simulink model "control_vectorial_dc"  (R2024b)
settings: Solver=ode14x  StartTime=0.0  StopTime=1  FixedStep=1e-6  MaxStep=1e-5  MinStep=1e-7  RelTol=1e-4  EnableMultiTasking=on
model workspace (MAT data in the model file):
  I_speed = 0.006
  P_flux = 0.72
  P_speed = 1.04
  P_torque = 0.72
  w = 2000
libraries: ee_lib x10, nesl_utility x7, fl_lib x5, eePwmGenerator x1, eeDcCurrentController x1, slpidlib x1
Description:
  | Field-Oriented Control al unui motor de tip Brushless DC, implementat cu uController, generator de PWM si driver.
settings Model: SimulationMode=accelerator  Creator=radu  LastModifiedBy=radu
settings SolverCC: PositivePriorityOrder=on  AutoInsertRateTranBlk=on
settings OptimizationCC: DefaultParameterBehavior=Inlined  EnhancedBackFolding=on  PassReuseOutputArgsThreshold=0  MaxStackSize=64  OptimizeBlockOrder=speed  DifferentSizesBufferReuse=on  OptimizationCustomize=off
settings DebuggingCC: ParameterTunabilityLossMsg=error
settings HardwareCC: HardwareBoardFeatureSet=SoCBlockset
settings ModelReferenceCC: ModelReferenceNumInstancesAllowed=Single
settings SFSimCC: MATLABDynamicMemAlloc=off
settings CodeAppCC: ForceParamTrailComments=on  OperatorAnnotations=on
settings GRTTargetCC: TargetLangStandard=C89/C90 (ANSI)

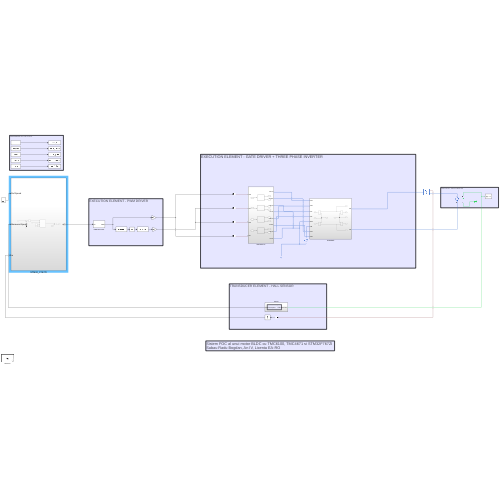
[thumbnail: Simulink's stored preview of the top-level diagram]
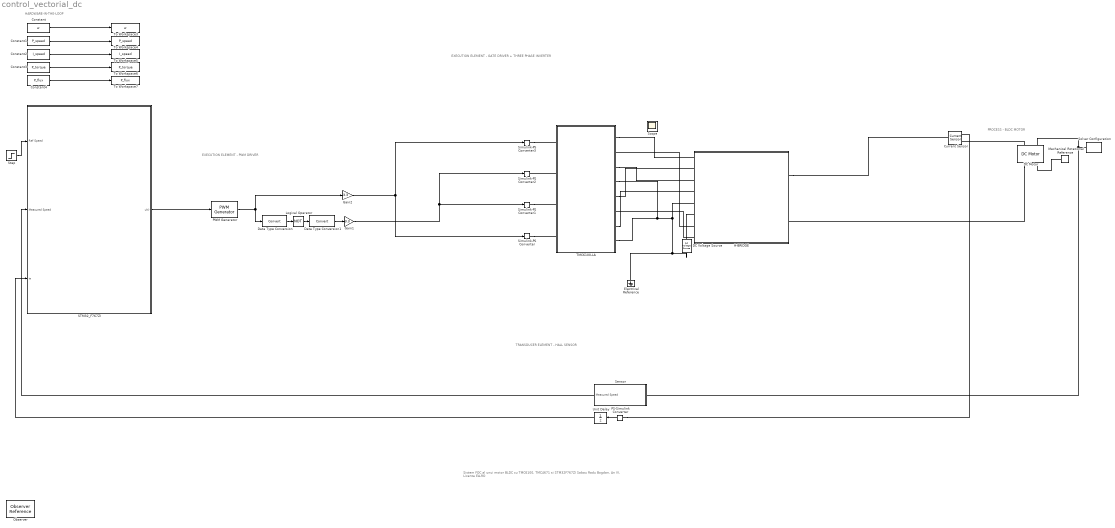
== system control_vectorial_dc ==
  note: HARDWARE-IN-THE-LOOP
  note: EXECUTION ELEMENT - PWM DRIVER
  note: PROCESS - BLDC MOTOR
  note: Sistem FOC al unui motor BLDC cu TMC6100, TMC4671 si STM32F767ZI
      | Sabau Radu Bogdan, An IV, Licenta EA-RO
  note: TRANSDUCER ELEMENT - HALL SENSOR
  note: EXECUTION ELEMENT - GATE DRIVER + THREE PHASE INVERTER
  Constant : Constant  Value=w
  Constant1 : Constant  Value=P_speed
  Constant2 : Constant  Value=I_speed
  Constant3 : Constant  Value=P_torque
  Constant4 : Constant  Value=P_flux
  Current Sensor : fl_lib/Electrical/Electrical Sensors/Current Sensor
  DC Motor : ee_lib/Electromechanical/Brushed Motors/DC Motor  field_option=ee.enum.field_option.pm  Rf=100 Ohm  Lf=1 H  Laf=0.15 H  If0=0 A  parameterization=ee.enum.dcparam_option.load_speed  Ra=3.9 Ohm  La=565e-6 H  emf_or_torque=ee.enum.emf_or_torque.kv  Kv=0.072e-3 V/rpm  Ki=6.876e-4 N*m/A  T_stall=0.24e-3 N*m  w_max=14974 rpm  w_rated=12850 rpm  P_rated=9.504 W  V_rated=12 V  lam_param=ee.enum.lam_param.damping  i_noload=0 A  V_i_noload=1.5 V  J=1e-6 kg*m^2  lam=5e-6 N*m*s/rad  speed0=0 rpm  t_fault_armature=1 s  t_fault_field=1 s  fault_action=simscape.enum.assert.action.none  alpha=3.93e-3 1/K  Tmeas=25 degC  thermal_mass=100 J/K  initial_temperature=25 degC
  DC Voltage Source : ee_lib/Additional Components/SPICE Sources/DC Voltage Source  DC=12 V
  Data Type Conversion : DataTypeConversion  SaturateOnIntegerOverflow=off  RndMeth=Floor
  Data Type Conversion1 : DataTypeConversion  SaturateOnIntegerOverflow=off  RndMeth=Floor
  Electrical Reference : fl_lib/Electrical/Electrical Elements/Electrical Reference
  Gain1 : Gain  Gain=3.3  OutDataTypeStr=double
  Gain2 : Gain  Gain=3.3  OutDataTypeStr=double
  H-BRIDGE : Subsystem
  Logical Operator : Logic  Operator=NOT  AllPortsSameDT=off  OutDataTypeStr=boolean
  Mechanical Rotational Reference : fl_lib/Mechanical/Rotational Elements/Mechanical Rotational Reference
  Observer : ObserverReference  ObserverModelName=control_vectorial_dc_v2_Observer1
  PS-Simulink Converter : nesl_utility/PS-Simulink Converter  PhysicalDomain=network_engine_domain  SubClassName=ps_output  LeftPortType=input  RightPortType=output  PseudoPeriodic=off  Frequencies=[]  VectorFormat=inherit  Unit=inherit  AffineConversion=off
  PWM Generator : eePwmGenerator/PWM Generator  CarrCount=Up  Tper=0.00002  Tdelay=0  Ts=1e-6
  STM32_F767ZI : Subsystem
  Sensor : Subsystem
  Simulink-PS Converter{,1..3} (4 alike) : nesl_utility/Simulink-PS Converter  PhysicalDomain=network_engine_domain  SubClassName=ps_input  LeftPortType=input  RightPortType=output  PseudoPeriodic=off  Frequencies=[]  NoiseDistribution=none  NoiseParameters=[]  Unit=1  AffineConversion=off  FilteringAndDerivatives=provide  SimscapeFilterOrder=1  InputFilterTimeConstant=0.001  UdotUserProvided=0
  Solver Configuration : nesl_utility/Solver Configuration  PhysicalDomain=network_engine_domain  SubClassName=solver  LeftPortType=input  RightPortType=generic  Tones=[]  Harmonics=[]  SimulateNoise=off  Profile=off  UseLocalSampling=off  EnableSwitchedLinearOptims=on  FrequencyDomain=off  UseCCode=off  RelTol=0.001  AbsTol=0.001  MinStep=1e-09  ToWorkspace=off  RevertToSquareIcSolve=off  NumHomotopyIterations=100  PhasorMode=off  PhasorModeNumHarmonics=1  ConsistencySolver=NEWTON_XTOL_AFTER_FTOL  IndexReductionMethod=DerivativeReplacement  DoDC=off  ResidualTolerance=1e-09  ConsistencyTolSource=GLOBAL  ConsistencyAbsTol=0.001  ConsistencyRelTol=0.001  ConsistencyTolFactor=1e-4  UseLocalSolver=on  LocalSolverChoice=NE_TRAPEZOIDAL_ADVANCER  ResolveIndetEquations=on  FunctionEvalNumThread=1  LocalSolverSampleTime=1e-6  DoFixedCost=on  MaxNonlinIter=3  MaxModeIter=2  ComputeImpulses=off  ImpulseIterations=2  LinearAlgebra=auto  LinearAlgebraNumThread=0  EquationFormulation=NE_TIME_EF  DelaysMemoryBudget=1024  AutomaticFiltering=on  FilteringTimeConstant=0.001  PartitionStorageMethod=AS_NEEDED  PartitionMemoryBudget=1024  PartitionMethod=ROBUST  MultibodyUseLocalSolver=off  MultibodyLocalSolverChoice=ODE1  MultibodyLocalSolverSampleTime=0.001
  Step : Step  Time=0  After=2500  SampleTime=1e-6
  TMC6100-LA : Subsystem
  To Workspace3 : ToWorkspace  VariableName=w  SaveFormat=Timeseries  SampleTime=-1
  To Workspace4 : ToWorkspace  VariableName=P_speed  SaveFormat=Timeseries  SampleTime=-1
  To Workspace5 : ToWorkspace  VariableName=I_speed  SaveFormat=Timeseries  SampleTime=-1
  To Workspace6 : ToWorkspace  VariableName=P_torque  SaveFormat=Timeseries  SampleTime=-1
  To Workspace7 : ToWorkspace  VariableName=P_flux  SaveFormat=Timeseries  SampleTime=-1
  Unit Delay : UnitDelay  SampleTime=-1  HasFrameUpgradeWarning=on
  Scope : Scope
  wires:
  Sensor/1(Measured Speed) -> STM32_F767ZI/2(Measured Speed)
  Step/1 -> STM32_F767ZI/1(Ref Speed)
  Constant/1 -> To Workspace3/1
  Constant4/1 -> To Workspace7/1
  Constant2/1 -> To Workspace5/1
  Constant3/1 -> To Workspace6/1
  Constant1/1 -> To Workspace4/1
  PWM Generator/1 -> Gain2/1, Data Type Conversion/1
  STM32_F767ZI/1(u(t)) -> PWM Generator/1
  Data Type Conversion/1 -> Logical Operator/1
  Data Type Conversion1/1 -> Gain1/1
  Logical Operator/1 -> Data Type Conversion1/1
  PS-Simulink Converter/1 -> Unit Delay/1
  Unit Delay/1 -> STM32_F767ZI/3(ia)
  Gain1/1 -> Simulink-PS Converter1/1, Simulink-PS Converter2/1
  Gain2/1 -> Simulink-PS Converter/1, Simulink-PS Converter3/1
  connections:
  Sensor/LConn1 -- Solver Configuration/RConn1 -- DC Motor/LConn2
  Mechanical Rotational Reference/LConn1 -- DC Motor/RConn2
  TMC6100-LA/RConn1 -- H-BRIDGE/LConn1
  TMC6100-LA/RConn3 -- H-BRIDGE/LConn3
  TMC6100-LA/RConn5 -- H-BRIDGE/LConn2
  TMC6100-LA/RConn7 -- H-BRIDGE/LConn4
  TMC6100-LA/RConn8 -- TMC6100-LA/RConn4 -- DC Voltage Source/RConn1 -- Electrical Reference/LConn1 -- H-BRIDGE/LConn5
  H-BRIDGE/LConn6 -- DC Voltage Source/LConn1
  Simulink-PS Converter3/RConn1 -- TMC6100-LA/LConn1
  TMC6100-LA/LConn2 -- Simulink-PS Converter2/RConn1
  Simulink-PS Converter1/RConn1 -- TMC6100-LA/LConn3
  Simulink-PS Converter/RConn1 -- TMC6100-LA/LConn4
  H-BRIDGE/LConn7 -- TMC6100-LA/RConn2
  H-BRIDGE/LConn8 -- TMC6100-LA/RConn6
  DC Motor/RConn1 -- H-BRIDGE/RConn2
  DC Motor/LConn1 -- Current Sensor/RConn2
  H-BRIDGE/RConn1 -- Current Sensor/LConn1
  PS-Simulink Converter/LConn1 -- Current Sensor/RConn1

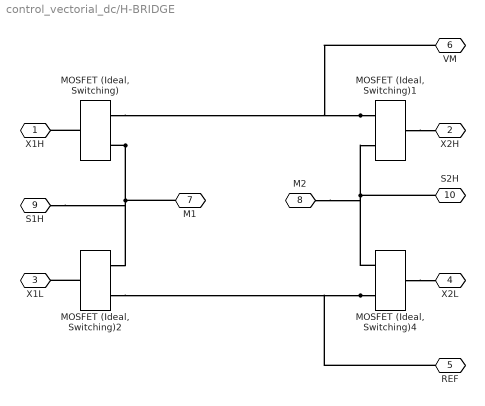
== system control_vectorial_dc/H-BRIDGE ==
  MOSFET (Ideal, Switching){,1..2,4} (4 alike) : ee_lib/Semiconductors & Converters/MOSFET (Ideal, Switching)  port_option=ee.enum.controlport.elec  Rds=0.0021 Ohm  Goff=140 1/Ohm  Vth=3 V  diode_param=ee.enum.semiconductors.protectionDiode.nodynamics  diode_Vf=0.1 V  diode_Ron=0.001 Ohm  diode_Goff=1e-5 1/Ohm  diode_C=50e-9 F  diode_iRM=-235 A  diode_iF=300 A  diode_idot=-50 A/us  diode_trr_param=ee.enum.converters.diodeReverseParam.trr_factor  diode_trr_factor=3  diode_trr=15 us  diode_Qrr=1500 s*uA  ids_specify=off  ids_priority=None  ids=0 A  ids_nominal_specify=off  ids_nominal_value=1  ids_nominal_unit=A  vds_specify=off  vds_priority=None  vds=0 V  vds_nominal_specify=off  vds_nominal_value=1  vds_nominal_unit=V  vgs_specify=off  vgs_priority=None  vgs=0 V  vgs_nominal_specify=off  vgs_nominal_value=1  vgs_nominal_unit=V  thermal_loss_option=ee.enum.converters.thermalLossOption.constantvalues  Von_data=[0, 1.8, 3.2, 6, 10, 16; 0, 2, 5.5, 9.5, 15, 25] V  Tj=[298.15, 448.15] K  Iout_data=[0, 20, 40, 60, 80, 100] A  Eon_data=[0, 55.04, 124.57, 235.53, 362.12; 0, 71.25, 161.25, 304.88, 468.75] * 1e-6 J  Eoff_data=[0, 18, 30, 56.1, 76.5; 0, 22.5, 37.5, 70.13, 95.63] * 1e-6 J  Eon_data_3D=[zeros(2, 5, 3)] J  Eoff_data_3D=[zeros(2, 5, 3)] J  Tj_loss=[298.15, 448.15] K  Iout_data_loss=[0, 10, 20, 30, 40] A  tabulateWithVds=false  Vds_loss=[0, 150, 300] V  Eon_scalar=22.86e-3 J  Eoff_scalar=17.14e-3 J  Voff=300 V  Iout_scalar=600 A  useCurrentFromPreviousCycle=false  useVoltageFromPreviousCycle=false  diodeModelType=ee.enum.converters.diodeModelType.pwl  diodeTableType=ee.enum.diode.tableType.IfMat  diode_ReverseIVType=ee.enum.diode.diodeReverseIV.constant  diode_IfMat=[.07, .12, .19, 1.75, 4.24, 7.32, 11.2; .16, .3, .72, 2.14, 4.02, 6.35, 9.12] A  diode_VfMat=[.9, 1.15, 1.25, 1.5, 1.75, 2.17, 2.6, 2.85; .58, .68, .75, 1.1, 1.38, 1.77, 2.27, 2.7] V  diode_TjVec=[25, 125] degC  diode_VfVec=[.5, .7, .9, 1.3, 1.7, 2.1, 2.5] V  diode_IfVec=[.1, .2, .5, 1, 2, 4, 7, 10] A  diode_IrMat=[1e-06, 2e-06, 5e-06, 1e-05, 2.5e-05, 5e-05, .0001; 2e-06, 5e-06, 1e-05, 4e-05, 8e-05, .0002, .0005] A  diode_VrMat=[10, 100, 200, 250, 300, 325, 350; 10, 70, 160, 220, 270, 300, 320] V  diode_VrVec=[10, 20, 40, 50, 70, 80, 100] V  diode_IrVec=[1e-06, 2e-06, 5e-06, 1e-05, 2e-05, 5e-05, .0001] A  diode_Vr=-600 V  diode_Ls=150 nH  diode_Erec=0.03 J  diode_rec_loss_model=ee.enum.diode.reverseRecoveryModel.fixed  diode_ErecVal=0 J  diode_scaleWithIandV=true  diode_ErecMat=zeros(2, 3) J  diode_TjrecVec=[298.15, 398.15] K  diode_IfrecVec=[.1, 1, 10] A  diode_IrecVal=10 A  diode_VrecVal=10 V  diode_tFilter=1 / 1000 / 100 s  separateThermalPortForDiode=false  thermal_network_parameterization=ee.enum.thermalNetworkTopology.external  Rth=[.03, .2] K/W  Rth_Cauer=[.03, .1, .2] K/W  Rth_Foster=[.08, .14, .22, .16] K/W  thermal_mass_parameterization=ee.enum.thermalNetwork.timeconstant  thermal_mass=[3, 25] J/K  thermal_mass_Cauer=[3, 10, 25] J/K  thermal_mass_Foster=[.001, .005, .05, .5] J/K  thermal_time_constant=[.1, 5] s  thermal_time_constant_Cauer=[.1, 1, 5] s  thermal_time_constant_Foster=[7e-05, .0007, .01, .08] s  thermal_mass_initial_temperatures=[25, 25] degC  thermal_mass_initial_temperatures_Cauer=[25, 25, 25] degC  junction_thermal_mass=0.1 J/K  Tvec_initial_Foster=[25, 25, 25, 25] degC  RthDiode=[.03, .2] K/W  RthCauerDiode=[.03, .1, .2] K/W  RthFosterDiode=[.03, .2] K/W  thermalMassDiode=[3, 25] J/K  thermalMassCauerDiode=[3, 10, 25] J/K  thermalMassFosterDiode=[33, 50] J/K  thermalTauDiode=[.1, 5] s  thermalTauCauerDiode=[.1, 1, 5] s  thermalTauFosterDiode=[1, 10] s  thermalMassInitTempDiode=[25, 25] degC  thermalMassInitTempCauerDiode=[25, 25, 25] degC  junctionthermalMassDiode=0.1 J/K  TVecInitialFosterDiode=[25, 25, 25, 25] degC  no_thermal_network=0  mosfet_junction_temperature_specify=off  mosfet_junction_temperature_priority=None  mosfet_junction_temperature=25 degC  mosfet_junction_temperature_nominal_specify=off  mosfet_junction_temperature_nominal_value=1  mosfet_junction_temperature_nominal_unit=degC  diode_junction_temperature_specify=off  diode_junction_temperature_priority=None  diode_junction_temperature=25 degC  diode_junction_temperature_nominal_specify=off  diode_junction_temperature_nominal_value=1  diode_junction_temperature_nominal_unit=degC  Qj_specify=off  Qj_priority=None  Qj=0 W  Qj_nominal_specify=off  Qj_nominal_value=1  Qj_nominal_unit=W  accumulatedSwitchingLosses_specify=off  accumulatedSwitchingLosses_priority=None  accumulatedSwitchingLosses=0 J
      settings: InternalSimscapePortConfiguration="{\"Bottom\":[],\"Left\":[{\"id\":\"G_elec\",\"label\":\"\",\"type\":\"foundation.electrical.electrical\"}],\"Right\":[{\"id\":\"D\",\"label\":\"\",\"type\":\"foundation.electrical.electrical\"},{\"id\":\"S\",\"label\":\"\",\"type\":\"foundation.electrical.electrical\"}],\"Top\":[]}"
  X1H : PMIOPort  Side=Left
  X2H : PMIOPort  Port=2  Side=Left
  X1L : PMIOPort  Port=3  Side=Left
  X2L : PMIOPort  Port=4  Side=Left
  REF : PMIOPort  Port=5  Side=Left
  VM : PMIOPort  Port=6  Side=Left
  M1 : PMIOPort  Port=7  Side=Right
  M2 : PMIOPort  Port=8  Side=Right
  S1H : PMIOPort  Port=9  Side=Left
  S2H : PMIOPort  Port=10  Side=Left
  connections:
  "MOSFET (Ideal, Switching)"/RConn2 -- S1H/RConn1 -- "MOSFET (Ideal, Switching)2"/RConn1 -- M1/RConn1
  "MOSFET (Ideal, Switching)4"/LConn1 -- X2L/RConn1
  "MOSFET (Ideal, Switching)4"/RConn2 -- "MOSFET (Ideal, Switching)2"/RConn2 -- REF/RConn1
  "MOSFET (Ideal, Switching)2"/LConn1 -- X1L/RConn1
  "MOSFET (Ideal, Switching)"/LConn1 -- X1H/RConn1
  "MOSFET (Ideal, Switching)1"/RConn1 -- "MOSFET (Ideal, Switching)"/RConn1 -- VM/RConn1
  "MOSFET (Ideal, Switching)1"/LConn1 -- X2H/RConn1
  "MOSFET (Ideal, Switching)4"/RConn1 -- M2/RConn1 -- S2H/RConn1 -- "MOSFET (Ideal, Switching)1"/RConn2

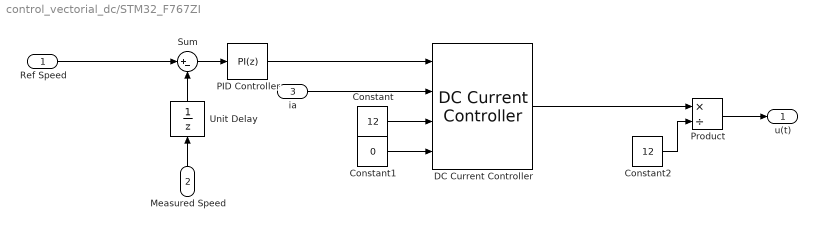
== system control_vectorial_dc/STM32_F767ZI ==
  Ref Speed : Inport
  Measured Speed : Inport  Port=2
  ia : Inport  Port=3
  Constant : Constant  Value=12
  Constant1 : Constant  Value=0
  Constant2 : Constant  Value=12
  DC Current Controller : eeDcCurrentController/DC Current Controller  Kp=1  Ki=1  Kaw=1  VoltLim=Positive and negative voltage  Ts=-1  Tsd=0.001  ActZC=off
      settings: LibrarySourceBlock=|
      | ee_sl_lib/General Machine
      | Control/DC Current Controller
  PID Controller : slpidlib/PID Controller  Controller=PI  Form=Parallel  TimeDomain=Discrete-time  UseExternalTs=off  SampleTime=1e-6  IntegratorMethod=Backward Euler  FilterMethod=Forward Euler  ControllerParametersSource=internal  P=P_speed  I=I_speed  UseKiTs=off  D=1  UseExternalDerivativeSource=off  N=100  UseFilter=on  TunerSelectOption=Transfer Function Based (PID Tuner App)  InitialConditionSource=internal  InitialConditionForIntegrator=0  InitialConditionForFilter=0  DifferentiatorICPrevScaledInput=0  ExternalReset=none  TrackingMode=off  Kt=1  LimitOutput=on  SatLimitsSource=internal  UpperSaturationLimit=15000  LowerSaturationLimit=-15000  LinearizeAsGain=on  AntiWindupMode=none  Kb=1  LimitIntegrator=off  UpperIntegratorSaturationLimit=inf  LowerIntegratorSaturationLimit=-inf  POutMin=[]  POutMax=[]  IOutMin=[]  IOutMax=[]  DOutMin=[]  DOutMax=[]  NOutMin=[]  NOutMax=[]  SumOutMin=[]  SumOutMax=[]  SaturationOutMin=[]  SaturationOutMax=[]  PParamMin=[]  PParamMax=[]  IParamMin=[]  IParamMax=[]  DParamMin=[]  DParamMax=[]  NParamMin=[]  NParamMax=[]  KbParamMin=[]  KbParamMax=[]  KtParamMin=[]  KtParamMax=[]  KbOutMin=[]  KbOutMax=[]  KtOutMin=[]  KtOutMax=[]  IntegratorOutMin=[]  IntegratorOutMax=[]  FilterOutMin=[]  FilterOutMax=[]  SumI1OutMin=[]  SumI1OutMax=[]  SumI2OutMin=[]  SumI2OutMax=[]  SumI3OutMin=[]  SumI3OutMax=[]  SumI4OutMin=[]  SumI4OutMax=[]  SumDOutMin=[]  SumDOutMax=[]  DifferentiatorOutMin=[]  DifferentiatorOutMax=[]  FilterDiffOutCoefMin=[]  FilterDiffOutCoefMax=[]  ReciprocalOutMin=[]  ReciprocalOutMax=[]  SumDenOutMin=[]  SumDenOutMax=[]  SumNumOutMin=[]  SumNumOutMax=[]  DivideOutMin=[]  DivideOutMax=[]  UdiffTsProdOutMin=[]  UdiffTsProdOutMax=[]  NTsProdOutMin=[]  NTsProdOutMax=[]  UintegralTsProdOutMin=[]  UintegralTsProdOutMax=[]  UngainTsProdOutMin=[]  UngainTsProdOutMax=[]  ClampingZeroOutDataTypeStr=Inherit: Inherit via back propagation  ClampingZeroOutMin=[]  ClampingZeroOutMax=[]  FilterDenConstantOutDataTypeStr=Inherit: Inherit via back propagation  FilterDenConstantOutMin=[]  FilterDenConstantOutMax=[]  PCopyOutDataTypeStr=Inherit: Inherit via back propagation  PCopyOutMin=[]  PCopyOutMax=[]  NCopyOutDataTypeStr=Inherit: Inherit via back propagation  NCopyOutMin=[]  NCopyOutMax=[]  IntegratorContinuousStateAttributes=''  IntegratorStateMustResolveToSignalObject=off  IntegratorRTWStateStorageClass=Auto  FilterContinuousStateAttributes=''  FilterStateMustResolveToSignalObject=off  FilterRTWStateStorageClass=Auto  ParallelPVariant=InternalParameters  IdealPVariant=Disabled  IVariant=InternalParameters  DVariant=Disabled  IntegratorVariant=Discrete  SatVariant=Enabled  AWVariant=Passthrough  PCopyVariant=Disabled  TRVariant=Disabled  FdbkBlocksVariant=Forward  IdealPFdbkVariant=Disabled  SatFdbkVariant=Disabled  DerivativeFilterVariant=Disabled  NVariant=Disabled  NCopyVariant=Disabled_SignalSpec  FilterICVariant=Disabled  IntegratorICVariant=InternalICs  ExternalResetVariant=Disabled  TRSumVariant=Passthrough  SumFdbkVariant=Disabled  SumVariant=Sum_PI  TsampFilterVariant=InternalTs  TsampNgainVariant=Passthrough  TsampIntegralVariant=Disabled_SignalSpec  ExternalSaturationOutDataTypeStr=Inherit: Same as second input  DerivativeSourceVariant=Disabled  PreIntVariant=InternalPreInt
  Product : Product  Inputs=*/
  Sum : Sum  Inputs=|+-
  Unit Delay : UnitDelay  SampleTime=1e-5  HasFrameUpgradeWarning=on
  u(t) : Outport
  wires:
  Sum/1 -> PID Controller/1
  Ref Speed/1 -> Sum/1
  Unit Delay/1 -> Sum/2
  Measured Speed/1 -> Unit Delay/1
  Product/1 -> u(t)/1
  Constant2/1 -> Product/2
  Constant1/1 -> DC Current Controller/4
  Constant/1 -> DC Current Controller/3
  DC Current Controller/1 -> Product/1
  ia/1 -> DC Current Controller/2
  PID Controller/1 -> DC Current Controller/1

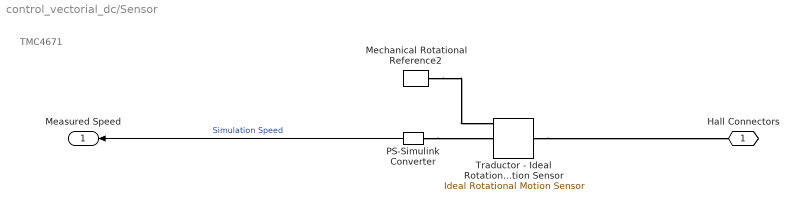
== system control_vectorial_dc/Sensor ==
  note: TMC4671
  Mechanical Rotational Reference2 : fl_lib/Mechanical/Rotational Elements/Mechanical Rotational Reference
  PS-Simulink Converter : nesl_utility/PS-Simulink Converter  PhysicalDomain=network_engine_domain  SubClassName=ps_output  LeftPortType=input  RightPortType=output  PseudoPeriodic=off  Frequencies=[]  VectorFormat=inherit  Unit=rpm  AffineConversion=off
  Traductor - Ideal Rotational Motion Sensor : fl_lib/Mechanical/Mechanical Sensors/Ideal Rotational Motion Sensor  reference=foundation.enum.MeasurementReference.difference  acceleration_port=false  velocity_port=true  position_port=true  wrap_angle=false  offset=0 deg
  Hall Connectors : PMIOPort  Side=Left
  Measured Speed : Outport
  wires:
  PS-Simulink Converter/1 -> Measured Speed/1  "Simulation Speed"
  connections:
  PS-Simulink Converter/LConn1 -- Traductor - Ideal Rotational Motion Sensor/RConn2
  Mechanical Rotational Reference2/LConn1 -- Traductor - Ideal Rotational Motion Sensor/RConn1
  Traductor - Ideal Rotational Motion Sensor/LConn1 -- Hall Connectors/RConn1

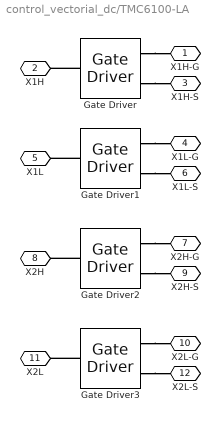
== system control_vectorial_dc/TMC6100-LA ==
  Gate Driver{,1..3} (4 alike) : ee_lib/Semiconductors & Converters/Gate Driver  port_option=ee.enum.controlport.ps  uHigh=2.0 V  uLow=0.8 V  uHighValue=2.31  uLowValue=0.99  vHigh=12 V  vLow=0 V  tHigh=85 ns  tLow=85 ns  parameterization=ee.enum.semiconductors.gateDriverParam.riseAndFallTimes  rHigh=2 Ohm  rLow=2 Ohm  tRise=10 ns  tFall=10 ns  cLoad=10 nF  t_fault=1 s  ZonTime_specify=off  ZonTime_priority=None  ZonTime=0 s  ZoffTime_specify=off  ZoffTime_priority=None  ZoffTime=0 s
      settings: InternalSimscapePortConfiguration="{\"Bottom\":[],\"Left\":[{\"id\":\"u\",\"label\":\"u\",\"type\":\"input\"}],\"Right\":[{\"id\":\"G\",\"label\":\"G\",\"type\":\"foundation.electrical.electrical\"},{\"id\":\"S\",\"label\":\"S\",\"type\":\"foundation.electrical.electrical\"}],\"Top\":[]}"
  X1H-G : PMIOPort  Side=Right
  X1H : PMIOPort  Port=2  Side=Left
  X1H-S : PMIOPort  Port=3  Side=Right
  X1L-G : PMIOPort  Port=4  Side=Right
  X1L : PMIOPort  Port=5  Side=Left
  X1L-S : PMIOPort  Port=6  Side=Right
  X2H-G : PMIOPort  Port=7  Side=Right
  X2H : PMIOPort  Port=8  Side=Left
  X2H-S : PMIOPort  Port=9  Side=Right
  X2L-G : PMIOPort  Port=10  Side=Right
  X2L : PMIOPort  Port=11  Side=Left
  X2L-S : PMIOPort  Port=12  Side=Right
  connections:
  Gate Driver2/LConn1 -- X2H/RConn1
  Gate Driver1/LConn1 -- X1L/RConn1
  Gate Driver1/RConn1 -- X1L-G/RConn1
  Gate Driver1/RConn2 -- X1L-S/RConn1
  Gate Driver2/RConn1 -- X2H-G/RConn1
  Gate Driver/RConn2 -- X1H-S/RConn1
  Gate Driver3/LConn1 -- X2L/RConn1
  Gate Driver3/RConn2 -- X2L-S/RConn1
  Gate Driver3/RConn1 -- X2L-G/RConn1
  Gate Driver/RConn1 -- X1H-G/RConn1
  Gate Driver2/RConn2 -- X2H-S/RConn1
  Gate Driver/LConn1 -- X1H/RConn1
